simulink model "task11_simulink"  (R2023a)
settings: Solver=ode45  StartTime=0  StopTime=20  RelTol=1e-3  EnableMultiTasking=on
model workspace (MAT data in the model file):
  op_snapshot1 = opcond.OperatingPoint
  op_snapshot1.Model_ = 'plant_ToBeCompletedForTask7'
  op_snapshot1.Time_ = 10000
  op_snapshot1.States_(1) = opcond.StatePoint
  op_snapshot1.States_(1).Nx_ = 1
  op_snapshot1.States_(1).Block_ = 'plant_ToBeCompletedForTask7/plant/Integrator'
  op_snapshot1.States_(1).x_ = 352.0988
  op_snapshot1.States_(2) = opcond.StatePoint
  op_snapshot1.States_(2).Nx_ = 1
  op_snapshot1.States_(2).Block_ = 'plant_ToBeCompletedForTask7/plant/Integrator1'
  op_snapshot1.States_(2).x_ = 0.5
  op_snapshot1.States_(3) = opcond.StatePoint
  op_snapshot1.States_(3).Nx_ = 1
  op_snapshot1.States_(3).Block_ = 'plant_ToBeCompletedForTask7/MPC Controller/MPC/last_mv'
  op_snapshot1.States_(3).x_ = 301.5795
  op_snapshot1.States_(3).Ts_ = [0.1 0]
  op_snapshot1.States_(3).SampleType_ = 'DSTATE'
libraries: mpclib x1
settings Model: Creator=The MathWorks, Inc.  LastModifiedBy=xiong
settings SolverCC: AlgebraicLoopSolver=TrustRegion
settings DataIOCC: ExternalInput=getinputstruct(op_snapshot1)  LimitDataPoints=on  LoadExternalInput=on  SaveFormat=Array  SignalLoggingName=logsOut
settings OptimizationCC: BooleanDataType=off  DefaultParameterBehavior=Inlined  InlineInvariantSignals=on  BufferReuse=off  ExpressionDepthLimit=2147483647  InitFltsAndDblsToZero=on  LifeSpan=inf
settings DebuggingCC: SaveWithParameterizedLinksMsg=none  UnderspecifiedInitializationDetection=Classic  MergeDetectMultiDrivingBlocksExec=none  CheckExecutionContextPreStartOutputMsg=on  SignalResolutionControl=TryResolveAllWithWarning  MultiTaskDSMMsg=warning  MultiTaskCondExecSysMsg=none  UnconnectedInputMsg=warning  UnconnectedOutputMsg=warning  UnconnectedLineMsg=warning  StateNameClashWarn=warning  SFUnexpectedBacktrackingDiag=warning  SFNoUnconditionalDefaultTransitionDiag=warning  SFExecutionAtInitializationDiag=none  ArithmeticOperatorsInVariantConditions=warning
settings HardwareCC: ProdBitPerPointer=32  ProdBitPerSizeT=32  ProdBitPerPtrDiffT=32  ProdLargestAtomicFloat=None  ProdIntDivRoundTo=Undefined  ProdEndianess=Unspecified  ProdWordSize=32  ProdHWDeviceType=32-bit Generic  TargetUnknown=on
settings ModelReferenceCC: EnableRefExpFcnMdlSchedulingChecks=on  PropagateSignalLabelsOutOfModel=off
settings SFSimCC: SimUseLocalCustomCode=off  CustomCodeUndefinedFunction=UseInterfaceOnly
settings RTWCC: RTWUseLocalCustomCode=off  DLArmComputeVersion=19.05
settings CodeAppCC: StateflowObjectComments=on
settings GRTTargetCC: TargetFcnLib=ansi_tfl_tmw.mat  TargetLangStandard=C89/C90 (ANSI)  CombineOutputUpdateFcns=off  GRTInterface=on
settings ConfigComp: CovMetricSettings=dw  CovSaveCumulativeToWorkspaceVar=on  CovSaveSingleToWorkspaceVar=on  CovExternalEMLEnable=off  CovSFcnEnable=off

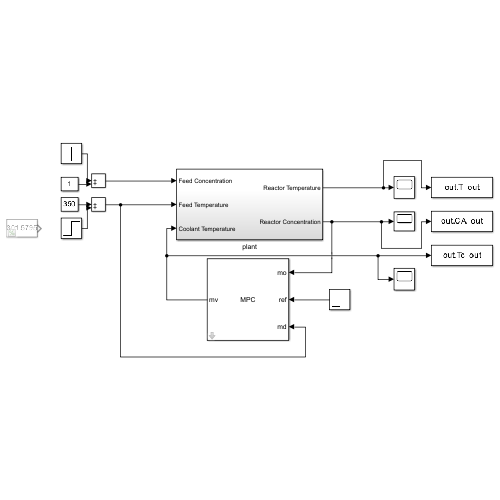
[thumbnail: Simulink's stored preview of the top-level diagram]
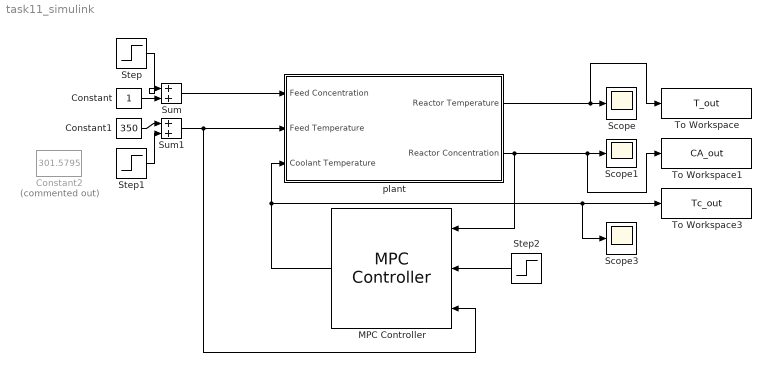
== system task11_simulink ==
  Constant : Constant
  Constant1 : Constant  Value=350
  Constant2 : Constant  Commented=on  Value=301.5795
  MPC Controller : mpclib/MPC Controller  SCDEnableBlockLinearizationSpecification=on  mpcobj=mpc1  is_multiple=0  enable_value=0  return_u0=off  updateMPCinCallerWorkspace=on  md_inport=on  mv_inport=off  uref_inport=off  return_cost=off  return_mvseq=off  return_qpstatus=off  return_xseq=off  return_state=off  return_ovseq=off  state_inport=off  umin_inport=off  umax_inport=off  ymin_inport=off  ymax_inport=off  cc_inport=off  ywt_inport=off  uwt_inport=off  duwt_inport=off  rhoeps_inport=off  pm_inport=off  MaximumP=10  HorizonChoice=FixedHorizon  n_ts=0.1  n_p=15  n_mv=1  n_md=1  n_ud=1  n_mo=1  n_uo=1  BlockDataType=double  SampleTimeInherited=off  switch_inport=off
  Scope : Scope
  Scope1 : Scope
  Scope3 : Scope
  Step : Step  Time=12  After=0.1  SampleTime=0.1
  Step1 : Step  Time=4  After=10  SampleTime=0.1
  Step2 : Step  Time=8  Before=[0.5 352.1]  After=[0.6 352.1]  SampleTime=0.1
  Sum : Sum  Inputs=|++
  Sum1 : Sum  Inputs=|++
  To Workspace : ToWorkspace  VariableName=T_out  SaveFormat=Timeseries  SampleTime=-1
  To Workspace1 : ToWorkspace  VariableName=CA_out  SaveFormat=Timeseries  SampleTime=-1
  To Workspace3 : ToWorkspace  VariableName=Tc_out  SaveFormat=Timeseries  SampleTime=-1
  plant : Subsystem
  wires:
  plant/1(Reactor Temperature) -> To Workspace/1, Scope/1
  Constant/1 -> Sum/2
  plant/2(Reactor Concentration) -> MPC Controller/1, To Workspace1/1, Scope1/1
  Step2/1 -> MPC Controller/2
  Sum/1 -> plant/1(Feed Concentration)
  Step/1 -> Sum/1
  Sum1/1 -> MPC Controller/3, plant/2(Feed Temperature)
  Constant1/1 -> Sum1/1
  Step1/1 -> Sum1/2
  MPC Controller/1 -> plant/3(Coolant Temperature), Scope3/1, To Workspace3/1

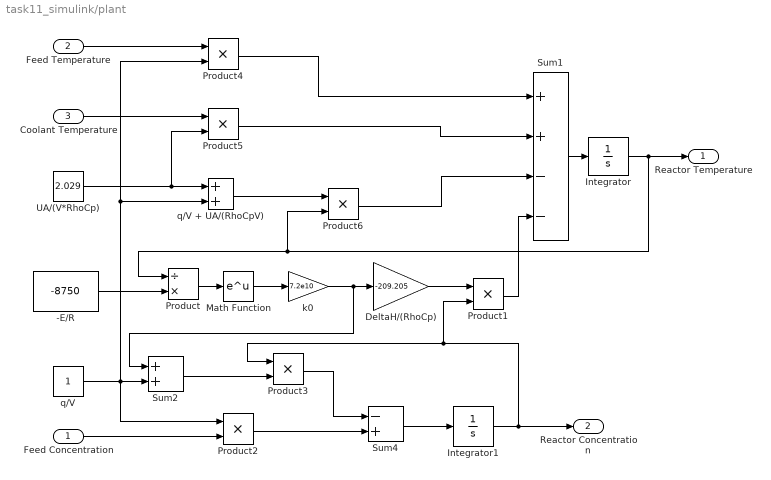
== system task11_simulink/plant ==
  Feed Concentration : Inport
  Feed Temperature : Inport  Port=2
  Coolant Temperature : Inport  Port=3
  -E/R : Constant  Value=-8750
  DeltaH/(RhoCp) : Gain  Gain=-209.205  SaturateOnIntegerOverflow=on  OutDataTypeStr=Inherit: Same as input  ParamDataTypeStr=Inherit: Same as input
  Integrator : Integrator  InitialCondition=352.0988  LimitOutput=on  LowerSaturationLimit=0
  Integrator1 : Integrator  InitialCondition=0.5  LimitOutput=on  LowerSaturationLimit=0
  Math Function : Math  SignedPower=on
  Product : Product  Inputs=/*  InputSameDT=on  RndMeth=Zero  SaturateOnIntegerOverflow=on  OutDataTypeStr=Inherit: Same as first input
  Product1 : Product  InputSameDT=on  RndMeth=Zero  SaturateOnIntegerOverflow=on  OutDataTypeStr=Inherit: Same as first input
  Product{2,4..6} (4 alike) : Product
  Product3 : Product  InputSameDT=on  RndMeth=Zero  SaturateOnIntegerOverflow=on  OutDataTypeStr=Inherit: Same as first input
  Sum1 : Sum  Inputs=++--  InputSameDT=on  SaturateOnIntegerOverflow=on  OutDataTypeStr=Inherit: Same as first input
  Sum2 : Sum  InputSameDT=on  SaturateOnIntegerOverflow=on  OutDataTypeStr=Inherit: Same as first input
  Sum4 : Sum  Inputs=-+  InputSameDT=on  SaturateOnIntegerOverflow=on  OutDataTypeStr=Inherit: Same as first input
  UA/(V*RhoCp) : Constant  Value=2.029
  k0 : Gain  Gain=7.2e10  SaturateOnIntegerOverflow=on  OutDataTypeStr=Inherit: Same as input  ParamDataTypeStr=Inherit: Same as input
  q/V : Constant
  q/V + UA/(RhoCpV) : Sum
  Reactor Temperature : Outport
  Reactor Concentration : Outport  Port=2
  wires:
  Product4/1 -> Sum1/1
  Sum1/1 -> Integrator/1
  Integrator/1 -> Product6/2, Product/1, Reactor Temperature/1
  Product5/1 -> Sum1/2
  Product6/1 -> Sum1/3
  Product/1 -> Math Function/1
  Math Function/1 -> k0/1
  DeltaH/(RhoCp)/1 -> Product1/1
  Product1/1 -> Sum1/4
  k0/1 -> DeltaH/(RhoCp)/1, Sum2/1
  -E/R/1 -> Product/2
  Product3/1 -> Sum4/1
  Sum4/1 -> Integrator1/1
  Integrator1/1 -> Product1/2, Product3/1, Reactor Concentration/1
  q/V/1 -> Product2/1, Sum2/2, Product4/2, q/V + UA/(RhoCpV)/2
  Product2/1 -> Sum4/2
  Feed Temperature/1 -> Product4/1
  Feed Concentration/1 -> Product2/2
  Coolant Temperature/1 -> Product5/1
  Sum2/1 -> Product3/2
  UA/(V*RhoCp)/1 -> Product5/2, q/V + UA/(RhoCpV)/1
  q/V + UA/(RhoCpV)/1 -> Product6/1
